simulink model "ThreephHW_diode"  (R2019a)
settings: Solver=VariableStepAuto  StartTime=0.0  StopTime=0.1  RelTol=1e-3
libraries: powerlib x22
settings Model: Creator=Amanna  LastModifiedBy=Amanna

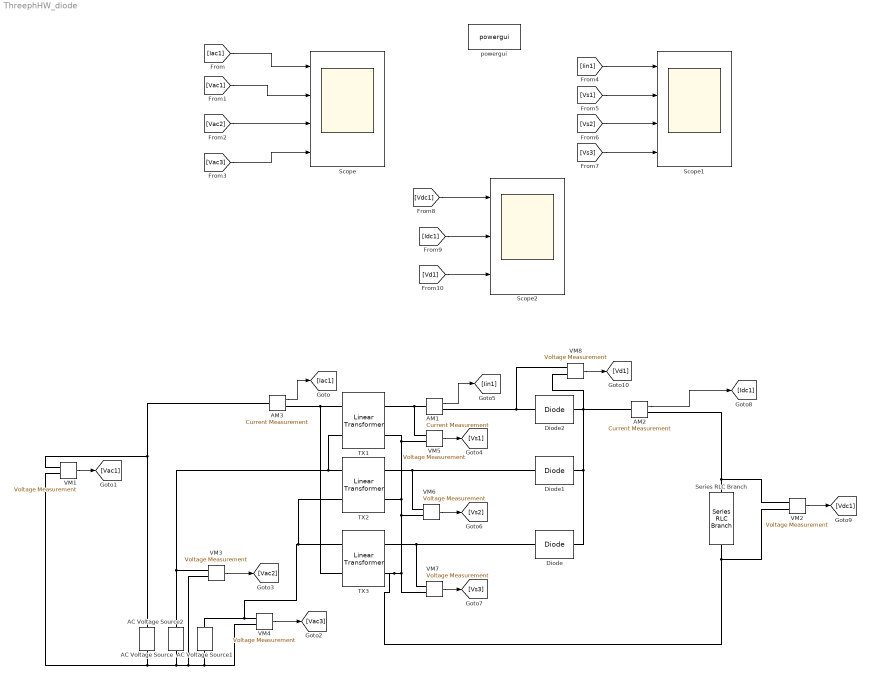
== system ThreephHW_diode ==
  AC Voltage Source : powerlib/Electrical Sources/AC Voltage Source  Amplitude=565.685  Phase=0  Frequency=50  SampleTime=0  Measurements=None  BusType=swing  Pref=10e3  Qref=0  Qmin=-inf  Qmax=+inf
      settings: SourceProductName=Simscape Electrical
  AC Voltage Source1 : powerlib/Electrical Sources/AC Voltage Source  Amplitude=565.685  Phase=-120  Frequency=50  SampleTime=0  Measurements=None  BusType=swing  Pref=10e3  Qref=0  Qmin=-inf  Qmax=+inf
      settings: SourceProductName=Simscape Electrical
  AC Voltage Source2 : powerlib/Electrical Sources/AC Voltage Source  Amplitude=565.685  Phase=120  Frequency=50  SampleTime=0  Measurements=None  BusType=swing  Pref=10e3  Qref=0  Qmin=-inf  Qmax=+inf
      settings: SourceProductName=Simscape Electrical
  AM1 : powerlib/Measurements/Current Measurement  PhasorSimulation=off  OutputType=Complex  PSBequivalent=0
      settings: SourceProductName=Simscape Electrical
  AM2 : powerlib/Measurements/Current Measurement  PhasorSimulation=off  OutputType=Complex  PSBequivalent=0
      settings: SourceProductName=Simscape Electrical
  AM3 : powerlib/Measurements/Current Measurement  PhasorSimulation=off  OutputType=Complex  PSBequivalent=0
      settings: SourceProductName=Simscape Electrical
  Diode : powerlib/Power Electronics/Diode  Ron=0.001  Lon=0  Vf=0.8  IC=0  UseSnubber=0  Rs=500  Cs=250e-9  Measurements=off
      settings: SourceProductName=Simscape Electrical
  Diode1 : powerlib/Power Electronics/Diode  Ron=0.001  Lon=0  Vf=0.8  IC=0  UseSnubber=0  Rs=500  Cs=250e-9  Measurements=off
      settings: SourceProductName=Simscape Electrical
  Diode2 : powerlib/Power Electronics/Diode  Ron=0.001  Lon=0  Vf=0.8  IC=0  UseSnubber=0  Rs=500  Cs=250e-9  Measurements=off
      settings: SourceProductName=Simscape Electrical
  Scope : Scope  NumInputPorts=4
  Scope1 : Scope  NumInputPorts=4
  Scope2 : Scope  NumInputPorts=3
  Series RLC Branch : powerlib/Elements/Series RLC Branch  LConnTagsString=__new0  RConnTagsString=__new0  BranchType=RL  Resistance=10  Inductance=10e-3  SetiL0=off  InitialCurrent=0  Capacitance=1e-6  Setx0=off  InitialVoltage=0  Measurements=None
      settings: SourceProductName=Simscape Electrical
  TX1 : powerlib/Elements/Linear Transformer  UNITS=pu  NominalPower=[ 250e6 50 ]  winding1="[ 600  0.002  0.08 ]"  winding2="[ 300  0.002  0.08 ]"  ThreeWindings=off  winding3=[ 315e3 0.002 0.08 ]  RmLm=[ 500 500 ]  Measurements=None  DataType=off
      settings: SourceProductName=Simscape Electrical
  TX2 : powerlib/Elements/Linear Transformer  UNITS=pu  NominalPower=[ 250e6 60 ]  winding1="[ 600  0.002  0.08 ]"  winding2="[ 300  0.002  0.08 ]"  ThreeWindings=off  winding3=[ 315e3 0.002 0.08 ]  RmLm=[ 500 500 ]  Measurements=None  DataType=off
      settings: SourceProductName=Simscape Electrical
  TX3 : powerlib/Elements/Linear Transformer  UNITS=pu  NominalPower=[ 250e6 60 ]  winding1="[ 600  0.002  0.08 ]"  winding2="[ 300  0.002  0.08 ]"  ThreeWindings=off  winding3=[ 315e3 0.002 0.08 ]  RmLm=[ 500 500 ]  Measurements=None  DataType=off
      settings: SourceProductName=Simscape Electrical
  VM{1..2,4..8} (7 alike) : powerlib/Measurements/Voltage Measurement  PhasorSimulation=off  OutputType=Complex  PSBequivalent=0
      settings: SourceProductName=Simscape Electrical
  "VM3 " : powerlib/Measurements/Voltage Measurement  PhasorSimulation=off  OutputType=Complex  PSBequivalent=0
      settings: SourceProductName=Simscape Electrical
  powergui : powerlib/powergui  Priority=1  SimulationMode=Continuous  SampleTime=50e-6  frequency=60  Iterations=50  frequencyindice=50  Pbase=100e6  ErrMax=1e-4  UnitsV=kV  UnitsW=MW  buscounter=0  FunctionMessages=off  echomessages=off  EnableUseOfTLC=off  CurrentSourceSwitches=off  DisableSnubberDevices=off  DisableRonSwitches=off  DisableVfSwitches=off  DisplayEquations=off  AutomaticDiscreteSolvers=off  SolverType=Tustin/Backward Euler (TBE)  Interpol=off  ExternalGateDelay=off  methode=off  Ts=100  x0status=blocks  SPID=on  SwTol=0  HookPort=off  NonlinearTolerance=0  nMaxIteration=15  ContinueOnMaxIteration=off  RestoreLinks=warning  ResistiveCurrentMeasurement=off  Frange=[0:2:500]  Ylog=off  Xlog=on  ShowGrid=off  save=off  variable=ZData  structure=0  ZoomFFT=off  StartTime=0.0  cycles=1  DisplayStyle=1  fundamental=60  FreqAxis=off  MaxFrequency=1000  frequencyindicesteady=1  RmsSteady=1  display=off
      settings: SourceProductName=Simscape Electrical
  wires:
  AM3/1 -> [Iac1]
  VM1/1 -> [Vac1]
  "VM3 "/1 -> [Vac2]
  VM4/1 -> [Vac3]
  VM5/1 -> [Vs1]
  AM1/1 -> [Iin1]
  VM6/1 -> [Vs2]
  VM7/1 -> [Vs3]
  AM2/1 -> [Idc1]
  VM2/1 -> [Vdc1]
  VM8/1 -> [Vd1]
  [Iac1] -> Scope/1
  [Vac1] -> Scope/2
  [Vac2] -> Scope/3
  [Vac3] -> Scope/4
  [Iin1] -> Scope1/1
  [Vs1] -> Scope1/2
  [Vs2] -> Scope1/3
  [Vs3] -> Scope1/4
  [Idc1] -> Scope2/2
  [Vdc1] -> Scope2/1
  [Vd1] -> Scope2/3
  connections:
  AM3/RConn1 -- TX3/LConn2 -- TX1/LConn1
  AC Voltage Source/LConn1 -- VM1/LConn2 -- AC Voltage Source2/LConn1 -- "VM3 "/LConn2 -- VM4/LConn2 -- AC Voltage Source1/LConn1
  VM4/LConn1 -- TX2/LConn2 -- TX3/LConn1 -- AC Voltage Source1/RConn1
  "VM3 "/LConn1 -- TX1/LConn2 -- TX2/LConn1 -- AC Voltage Source2/RConn1
  AC Voltage Source/RConn1 -- AM3/LConn1 -- VM1/LConn1
  AM1/LConn1 -- VM5/LConn1 -- TX1/RConn1
  Diode2/LConn1 -- VM8/LConn1 -- AM1/RConn1
  TX3/RConn2 -- VM2/LConn2 -- Series RLC Branch/RConn1 -- VM6/LConn2 -- VM5/LConn2 -- TX1/RConn2 -- TX2/RConn2 -- VM7/LConn2
  TX2/RConn1 -- Diode1/LConn1 -- VM6/LConn1
  Diode/LConn1 -- VM7/LConn1 -- TX3/RConn1
  Diode1/RConn1 -- Diode/RConn1 -- VM8/LConn2 -- AM2/LConn1 -- Diode2/RConn1
  AM2/RConn1 -- VM2/LConn1 -- Series RLC Branch/LConn1
